simulink model "SendUdp2Kinarm2021"  (R2021b)
settings: Solver=VariableStepAuto  StartTime=0.0  StopTime=5  FixedStep=0.1  RelTol=1e-3  EnableMultiTasking=on
values from neighbouring files (symbols this model uses):
  input = [XX(1,curr_time_idx),XX(2,curr_time_idx)]    [simulink_workflow.m]
undefined symbols (not defined in the file or in its folder): f
libraries: instrumentlib x6, slrealtimeutilitieslib x4, slrealtimeiplib x2, xcpprotocollib x1
settings Model: Creator=The MathWorks, Inc.  LastModifiedBy=willy
settings SolverCC: AlgebraicLoopSolver=TrustRegion
settings DataIOCC: LimitDataPoints=on  SaveFormat=Array  ReturnWorkspaceOutputs=off
settings OptimizationCC: ExpressionDepthLimit=2147483647  InitFltsAndDblsToZero=on  LifeSpan=inf
settings DebuggingCC: UnderspecifiedInitializationDetection=Classic  MergeDetectMultiDrivingBlocksExec=none  SolverPrmCheckMsg=warning  FcnCallInpInsideContextMsg=warning  StateNameClashWarn=warning  SFUnexpectedBacktrackingDiag=warning  SFNoUnconditionalDefaultTransitionDiag=warning  SFExecutionAtInitializationDiag=none  SFMachineParentedDataDiag=warning  ArithmeticOperatorsInVariantConditions=warning
settings HardwareCC: ProdBitPerPointer=32  ProdBitPerSizeT=32  ProdBitPerPtrDiffT=32  ProdLargestAtomicFloat=None  ProdIntDivRoundTo=Undefined  ProdEndianess=Unspecified  ProdWordSize=32  ProdHWDeviceType=32-bit Generic
settings ModelReferenceCC: PropagateSignalLabelsOutOfModel=off
settings SFSimCC: SimUseLocalCustomCode=off  CustomCodeUndefinedFunction=UseInterfaceOnly
settings RTWCC: RTWUseLocalCustomCode=off
settings CodeAppCC: StateflowObjectComments=on
settings GRTTargetCC: TargetFcnLib=ansi_tfl_tmw_new.mat  TargetLangStandard=C89/C90 (ANSI)  CombineOutputUpdateFcns=off  GRTInterface=on
settings ConfigComp: CovScope=ReferencedModels  CovMetricSettings=dw  CovSaveCumulativeToWorkspaceVar=on  CovSaveSingleToWorkspaceVar=on  CovExternalEMLEnable=off

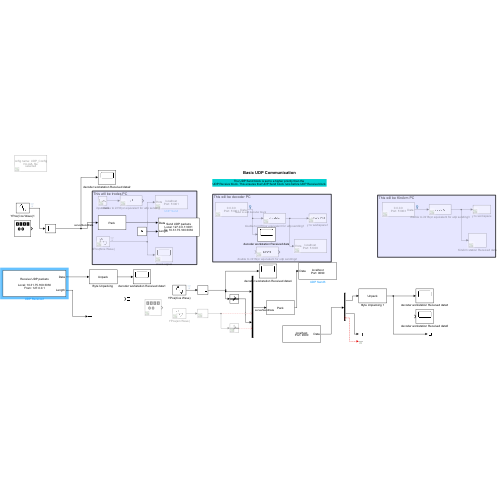
[thumbnail: Simulink's stored preview of the top-level diagram]
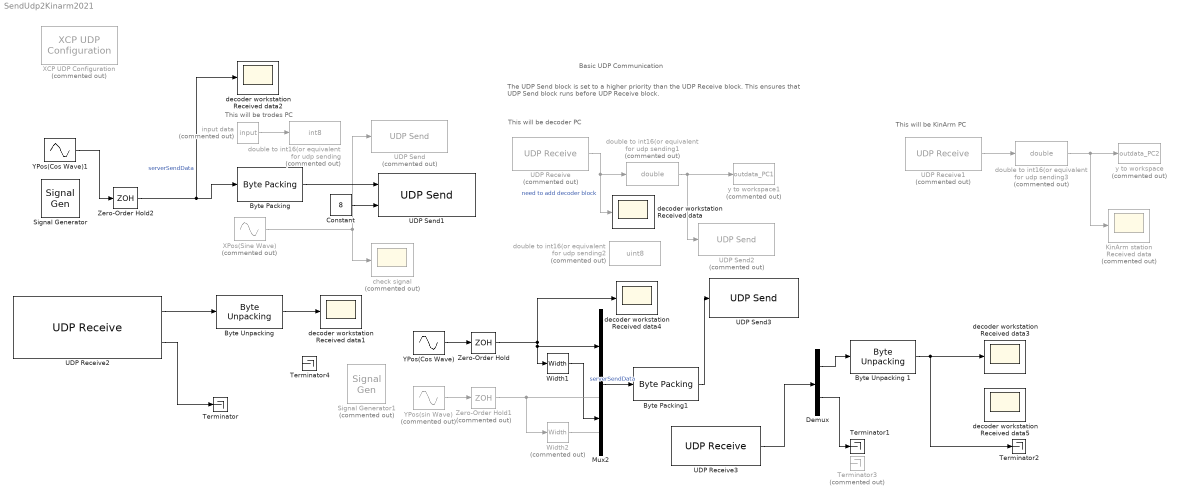
== system SendUdp2Kinarm2021 ==
  note: This will be KinArm PC
  note: This will be trodes PC
  note: This will be decoder PC
  note: The UDP Send block is set to a higher priority than the
      | UDP Receive block. This ensures that UDP Send block runs before UDP Receive block.
  note: Basic UDP Communication
  Byte Packing : slrealtimeutilitieslib/Byte Packing  MaskPackedDataType=uint8  MaskUnpackedDataTypes={'double'}  MaskAlignment=1
  Byte Packing1 : slrealtimeutilitieslib/Byte Packing  MaskPackedDataType=uint8  MaskUnpackedDataTypes={'double'}  MaskAlignment=1
  "Byte Unpacking " : slrealtimeutilitieslib/Byte Unpacking  MaskUnpackedDataTypes={'double'}  MaskUnpackedDataSizes={[1]}  MaskAlignment=1
      settings: SourceProductBaseCode=XP
  Byte Unpacking 1 : slrealtimeutilitieslib/Byte Unpacking  MaskUnpackedDataTypes={'double'}  MaskUnpackedDataSizes={[1]}  MaskAlignment=1
      settings: SourceProductBaseCode=XP
  Constant : Constant  Value=8
  Demux : Demux  Outputs=2
  KinArm station Received data : Scope  Commented=on
      settings: Priority=4
  Mux2 : Mux  Inputs=2
  Signal Generator : SignalGenerator  Frequency=0.5
  Signal Generator1 : SignalGenerator  Commented=on  WaveForm=square  Frequency=0.5
  Terminator{,1..2,4} (4 alike) : Terminator
  Terminator3 : Terminator  Commented=on
  UDP Receive : instrumentlib/UDP Receive  Priority=3  Commented=on  Host=localhost  Port=51000  LocalPort=51001  EnablePortSharing=off  GetLatestData=off  DataSize=[1 1]  DataType=double  ASCIIFormatting=%f,  Terminator=LF  ByteOrder=LittleEndian  EnableBlockingMode=on  Timeout=5  SampleTime=1  LocalAddress=0.0.0.0
  UDP Receive1 : instrumentlib/UDP Receive  Priority=3  Commented=on  Host=localhost  Port=51002  LocalPort=51003  EnablePortSharing=on  GetLatestData=off  DataSize=[1 1]  DataType=double  ASCIIFormatting=%f,  Terminator=LF  ByteOrder=BigEndian  EnableBlockingMode=on  Timeout=5  SampleTime=1  LocalAddress=0.0.0.0
  UDP Receive2 : slrealtimeiplib/UDP Receive  useHostTargetConn=off  ipAddress=10.31.75.160  localPort=3030  rcvWidth=8  rcvFmAny=off  fmAddress=127.0.0.1  sampleTime=0.01
      settings: SourceProductBaseCode=XP
  UDP Receive3 : instrumentlib/UDP Receive  Host=0.0.0.0  Port=8888  LocalPort=9090  EnablePortSharing=off  GetLatestData=off  DataSize=16  DataType=uint8  ASCIIFormatting=%f,  Terminator=LF  ByteOrder=BigEndian  EnableBlockingMode=on  Timeout=10  SampleTime=0.01  LocalAddress=localhost
  UDP Send : instrumentlib/UDP Send  Priority=2  Commented=on  Host=localhost  Port=51001  LocalPort=51000  EnablePortSharing=off  ByteOrder=LittleEndian  OutputDatagramPacketSize=1000  EnableBlockingMode=on  LocalAddress=0.0.0.0
  UDP Send1 : slrealtimeiplib/UDP Send  useHostTargetConn=off  toAddress=10.31.75.160  toPort=3030  sampleTime=0.01  ipAddress=127.0.0.1  localPort=3031
      settings: SourceProductBaseCode=XP
  UDP Send2 : instrumentlib/UDP Send  Priority=2  Commented=on  Host=localhost  Port=51003  LocalPort=51002  EnablePortSharing=on  ByteOrder=BigEndian  OutputDatagramPacketSize=512  EnableBlockingMode=on  LocalAddress=0.0.0.0
  UDP Send3 : instrumentlib/UDP Send  Host=localhost  Port=9090  LocalPort=8888  EnablePortSharing=off  ByteOrder=BigEndian  OutputDatagramPacketSize=16  EnableBlockingMode=on  LocalAddress=0.0.0.0
  Width1 : Width
  Width2 : Width  Commented=on
  XCP UDP Configuration : xcpprotocollib/UDP/XCP UDP Configuration  Priority=-100  Commented=on  SlaveName=UDP_Config1  SlaveID=1  EnableSecurity=off  EnableStatus=off  SampleTime=-1  HeaderErrDet=on  CTRScheme=One counter for all CTOs and DTOs  LocalAddress=auto  LocalPort=auto  DAQTimeout=Inf
      settings: SourceProductBaseCode=XP,VN
  XPos(Sine Wave) : Sin  Priority=1  Commented=on  SampleTime=0.1
  YPos(Cos Wave) : Sin  Priority=1  Phase=-0.5*pi
  YPos(Cos Wave)1 : Sin  Priority=1  Phase=-0.5*pi  SampleTime=0.01
  YPos(sin Wave) : Sin  Priority=1  Commented=on
  Zero-Order Hold : ZeroOrderHold  SampleTime=-1
  Zero-Order Hold1 : ZeroOrderHold  Commented=on  SampleTime=-1
  Zero-Order Hold2 : ZeroOrderHold  SampleTime=0.01
  check signal : Scope  Commented=on
      settings: Priority=4
  decoder workstation Received data{,1..5} (6 alike) : Scope
      settings: Priority=4
  double to int16(or equivalent for udp sending : DataTypeConversion  Commented=on  OutDataTypeStr=int8  RndMeth=Ceiling
  double to int16(or equivalent for udp sending1 : DataTypeConversion  Commented=on  OutDataTypeStr=double  RndMeth=Ceiling
  double to int16(or equivalent for udp sending2 : DataTypeConversion  Commented=on  OutDataTypeStr=uint8
  double to int16(or equivalent for udp sending3 : DataTypeConversion  Commented=on  OutDataTypeStr=double  RndMeth=Ceiling
  input data : Constant  Commented=on  Value=input
  y to workspace : ToWorkspace  Commented=on  VariableName=outdata_PC2  SampleTime=-1
      settings: Save2DSignal=2-D array (concatenate along first dimension)
  y to workspace1 : ToWorkspace  Commented=on  VariableName=outdata_PC1  SampleTime=1
      settings: Save2DSignal=2-D array (concatenate along first dimension)
  wires:
  XPos(Sine Wave)/1 -> UDP Send/1, check signal/1
  UDP Receive/1 -> double to int16(or equivalent for udp sending1/1, decoder workstation Received data/1  "need to add decoder block"
  input data/1 -> double to int16(or equivalent for udp sending/1
  UDP Receive1/1 -> double to int16(or equivalent for udp sending3/1
  double to int16(or equivalent for udp sending1/1 -> y to workspace1/1, UDP Send2/1
  double to int16(or equivalent for udp sending3/1 -> KinArm station Received data/1, y to workspace/1
  UDP Receive2/2 -> Terminator/1
  Constant/1 -> UDP Send1/2
  Width1/1 -> Mux2/2
  Mux2/1 -> Byte Packing1/1  "serverSendData"
  Byte Unpacking 1/1 -> Terminator2/1, decoder workstation Received data3/1
  Demux/1 -> Byte Unpacking 1/1
  Byte Packing1/1 -> UDP Send3/1
  UDP Receive3/1 -> Demux/1
  YPos(Cos Wave)/1 -> Zero-Order Hold/1
  Zero-Order Hold/1 -> Mux2/1, Width1/1, decoder workstation Received data4/1
  Width2/1 -> ?
  YPos(sin Wave)/1 -> Zero-Order Hold1/1
  Zero-Order Hold1/1 -> Width2/1
  Demux/2 -> Terminator1/1
  ? -> Terminator3/1
  Zero-Order Hold2/1 -> Byte Packing/1, decoder workstation Received data2/1  "serverSendData"
  Byte Packing/1 -> UDP Send1/1
  UDP Receive2/1 -> "Byte Unpacking "/1
  "Byte Unpacking "/1 -> decoder workstation Received data1/1
  YPos(Cos Wave)1/1 -> Zero-Order Hold2/1
